simulink model "matlab_file_rl"  (R2018a)
settings: Solver=FixedStepAuto  StartTime=0.0  StopTime=1  RelTol=1e-3
libraries: androiduilib x4
settings Model: Creator=akshay  LastModifiedBy=akshay
settings DataIOCC: LimitDataPoints=on  MaxDataPoints=5000
settings OptimizationCC: EnhancedBackFolding=on  PassReuseOutputArgsAs=Individual arguments  MaxStackSize=64  OptimizeBlockOrder=speed  DifferentSizesBufferReuse=on  OptimizationCustomize=off
settings DebuggingCC: ParameterTunabilityLossMsg=error
settings HardwareCC: ProdBitPerPointer=32  ProdBitPerSizeT=32  ProdBitPerPtrDiffT=32  ProdLargestAtomicInteger=Long  ProdLargestAtomicFloat=Double  ProdWordSize=32  ProdHWDeviceType=ARM Compatible->ARM Cortex
settings SFSimCC: MATLABDynamicMemAlloc=off
settings RTWCC: SystemTargetFile=ert.tlc  HardwareBoard=Android Device  TLCOptions="-aInlineSetEventsForThisBaseRateFcn=TLC_FALSE -aSuppressMultiTaskScheduler=TLC_FALSE  -aRateBasedStepFcn=0"  TemplateMakefile=ert_default_tmf  GenerateReport=on  RTWVerbose=off  Toolchain=Android SDK/NDK Tools  BuildConfiguration=Faster Runs  IncludeHyperlinkInReport=on  LaunchReport=on  GenerateTraceInfo=on  GenerateTraceReport=on  GenerateTraceReportSl=on  GenerateTraceReportSf=on  GenerateTraceReportEml=on
settings CodeAppCC: ForceParamTrailComments=on  IgnoreCustomStorageClasses=off  OperatorAnnotations=on  SimulinkDataObjDesc=on  SFDataObjDesc=on  InsertBlockDesc=on

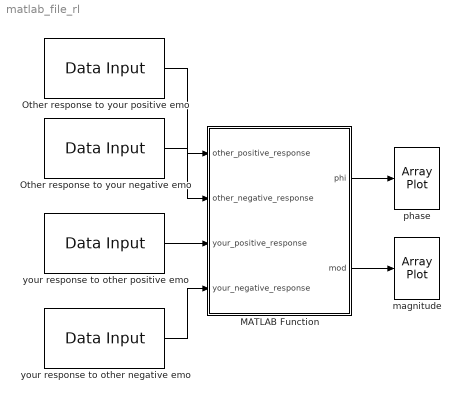
== system matlab_file_rl ==
  MATLAB Function : MATLAB Function  TreatAsAtomicUnit=on
  Other response to your negative emo : androiduilib/Data Input  isCharVector=off  Value=1  CharVector=Hello World  OutputDataType=double  maxCharVectorSize=100  DataInputId=matlab_file_rl/Other_response_to_your_negative_emo  SampleTime=0.1
      settings: SourceProductName=Simulink Support Package for Android Devices  SourceProductBaseCode=ANDROID
  Other response to your positive emo : androiduilib/Data Input  isCharVector=off  Value=1  CharVector=Hello World  OutputDataType=double  maxCharVectorSize=100  DataInputId=matlab_file_rl/Other_response_to_your_positive_emo  SampleTime=0.1
      settings: SourceProductName=Simulink Support Package for Android Devices  SourceProductBaseCode=ANDROID
  magnitude : ArrayPlot
  phase : ArrayPlot
  your response to other negative emo : androiduilib/Data Input  isCharVector=off  Value=1.0  CharVector=Hello World  OutputDataType=double  maxCharVectorSize=100  DataInputId=matlab_file_rl/your_response_to_other_negative_emo  SampleTime=0.1
      settings: SourceProductName=Simulink Support Package for Android Devices  SourceProductBaseCode=ANDROID
  your response to other positive emo : androiduilib/Data Input  isCharVector=off  Value=1.0  CharVector=Hello World  OutputDataType=double  maxCharVectorSize=100  DataInputId=matlab_file_rl/your_response_to_other_positive_emo  SampleTime=0.1
      settings: SourceProductName=Simulink Support Package for Android Devices  SourceProductBaseCode=ANDROID
  wires:
  Other response to your negative emo/1 -> MATLAB Function/2(other_negative_response)
  Other response to your positive emo/1 -> MATLAB Function/1(other_positive_response)
  your response to other positive emo/1 -> MATLAB Function/3(your_positive_response)
  your response to other negative emo/1 -> MATLAB Function/4(your_negative_response)
  MATLAB Function/1(phi) -> phase/1
  MATLAB Function/2(mod) -> magnitude/1

== matlab function matlab_file_rl/MATLAB Function ==
  data: other_positive_response input; phi output; other_negative_response input; your_positive_response input; your_negative_response input; mod output
function [phi, mod]  = rl_relation(other_positive_response,other_negative_response,...
    your_positive_response,your_negative_response)
[x,y] = meshgrid(-8:0.2:8,-8:0.2:8);
% asking question
% explain behavior of partner
% logic questions
% other_positive_response=input('others reponse to your positive feeling');
% other_negative_response=input('others reponse to your negative feeling');
% your_positive_response= input('your response to others positive feeling');
% your_negative_response= input('your response to others negative feeling');
% 2^4 functions


% 1 represents + ve emotions
% u= x
% v=y
% 0000 0001 0010 0011 0100 0101 0110 0111 1000 1001 1010 1011 1100 1101 1110 1111
%1 1111
if other_positive_response ==1 && other_negative_response== 1 &&...
your_positive_response== 1 && your_negative_response==1
u= y.^2;
v= x.^2;
w= u+j.*v;
out_1=reshape(u,length(u)*length(u),1);
out_2=reshape(v,length(v)*length(v),1);
out=reshape(w,length(w)*length(w),1);
phi= rad2deg(angle(out));
mod= abs(out);
%2 1110
elseif other_positive_response ==1 && other_negative_response== 1 &&...
your_positive_response== 1 && your_negative_response==0
u= y.^3;
v= x.^2;
w= u+j.*v;
out_1=reshape(u,length(u)*length(u),1);
out_2=reshape(v,length(v)*length(v),1);
out=reshape(w,length(w)*length(w),1);  
phi= rad2deg(angle(out));
mod= abs(out);    
%3 1101
elseif other_positive_response ==1 && other_negative_response== 1 &&...
your_positive_response== 0 && your_negative_response==1
u= -y.^3;
v= x.^2;
w= u+j.*v;
out_1=reshape(u,length(u)*length(u),1);
out_2=reshape(v,length(v)*length(v),1);
out=reshape(w,length(w)*length(w),1);
phi= rad2deg(angle(out));
mod= abs(out);
%4 1100
elseif other_positive_response ==1 && other_negative_response== 1 &&...
your_positive_response== 0 && your_negative_response==0
u= -y.^2;
v= x.^2;
w= u+j.*v;
out_1=reshape(u,length(u)*length(u),1);
out_2=reshape(v,length(v)*length(v),1);
out=reshape(w,length(w)*length(w),1);
phi= rad2deg(angle(out));
mod= abs(out);
%5 1011
elseif other_positive_response ==1 && other_negative_response== 0 &&...
your_positive_response== 1 && your_negative_response==1
u= y.^2;
v= x.^3;
w= u+j.*v;
out_1=reshape(u,length(u)*length(u),1);
out_2=reshape(v,length(v)*length(v),1);
out=reshape(w,length(w)*length(w),1);
phi= rad2deg(angle(out));
mod= abs(out);
%6 1010
elseif other_positive_response ==1 && other_negative_response== 0 &&...
your_positive_response== 1 && your_negative_response==0
u= y.^3;
v= x.^3;
w= u+j.*v;
out_1=reshape(u,length(u)*length(u),1);
out_2=reshape(v,length(v)*length(v),1);
out=reshape(w,length(w)*length(w),1);
phi= rad2deg(angle(out));
mod= abs(out);
%7 1001 other respond positive to your positive & negative to negative
% you respond -ve to their +ve and +ve to their -ve 
elseif other_positive_response ==1 && other_negative_response== 0 &&...
your_positive_response== 0 && your_negative_response==1
u= -y.^3;
v= x.^3;
w= u+j.*v;
out_1=reshape(u,length(u)*length(u),1);
out_2=reshape(v,length(v)*length(v),1);
out=reshape(w,length(w)*length(w),1);
phi= rad2deg(angle(out));
mod= abs(out);
% 8 1000
elseif other_positive_response ==1 && other_negative_response== 0 &&...
your_positive_response== 0 && your_negative_response==0
u= -y.^2;
v= x.^3;
w= u+j.*v;
out_1=reshape(u,length(u)*length(u),1);
out_2=reshape(v,length(v)*length(v),1);
out=reshape(w,length(w)*length(w),1);
phi= rad2deg(angle(out));
mod= abs(out);
%9 0111
elseif other_positive_response ==0 && other_negative_response== 1 &&...
your_positive_response==1 && your_negative_response==1
u= +y.^2;
v= -x.^3;
w= u+j.*v;
out_1=reshape(u,length(u)*length(u),1);
out_2=reshape(v,length(v)*length(v),1);
out=reshape(w,length(w)*length(w),1);
phi= rad2deg(angle(out));
mod= abs(out);
%10 0110
elseif other_positive_response ==0 && other_negative_response== 1 &&...
your_positive_response== 1 && your_negative_response==0
u= y.^3;
v= -x.^3;
w= u+j.*v;
out_1=reshape(u,length(u)*length(u),1);
out_2=reshape(v,length(v)*length(v),1);
out=reshape(w,length(w)*length(w),1);
phi= rad2deg(angle(out));
mod= abs(out);
% 11 0101
elseif other_positive_response ==0 && other_negative_response== 1 &&...
your_positive_response== 0 && your_negative_response==1
u= -y.^3;
v= -x.^3;
w= u+j.*v;
out_1=reshape(u,length(u)*length(u),1);
out_2=reshape(v,length(v)*length(v),1);
out=reshape(w,length(w)*length(w),1);
phi= rad2deg(angle(out));
mod= abs(out);
% 12 0100
elseif other_positive_response ==0 && other_negative_response== 1 &&...
your_positive_response== 0 && your_negative_response==0
u= -y.^2;
v= -x.^3;
w= u+j.*v;
out_1=reshape(u,length(u)*length(u),1);
out_2=reshape(v,length(v)*length(v),1);
out=reshape(w,length(w)*length(w),1);
phi= rad2deg(angle(out));
mod= abs(out);
% 13 0011
elseif other_positive_response ==0 && other_negative_response== 0 &&...
your_positive_response== 1 && your_negative_response==1
u= y.^2;
v= -x.^2;
w= u+j.*v;
out_1=reshape(u,length(u)*length(u),1);
out_2=reshape(v,length(v)*length(v),1);
out=reshape(w,length(w)*length(w),1);
phi= rad2deg(angle(out));
mod= abs(out);
% 14 0010
elseif other_positive_response ==0 && other_negative_response==0 &&...
your_positive_response== 1 && your_negative_response==0
u= y.^3;
v= -x.^2;
w= u+j.*v;
out_1=reshape(u,length(u)*length(u),1);
out_2=reshape(v,length(v)*length(v),1);
out=reshape(w,length(w)*length(w),1);
phi= rad2deg(angle(out));
mod= abs(out);
% 15 0001
elseif other_positive_response ==0 && other_negative_response== 0 &&...
your_positive_response== 0 && your_negative_response==1
u= -y.^3;
v= -x.^2;
w= u+j.*v;
out_1=reshape(u,length(u)*length(u),1);
out_2=reshape(v,length(v)*length(v),1);
out=reshape(w,length(w)*length(w),1);
phi= rad2deg(angle(out));
mod= abs(out);
% 16 0000
elseif other_positive_response ==0 && other_negative_response== 0 &&...
your_positive_response== 0 && your_negative_response==0
u= -y.^2;
v= -x.^2;
w= u+j.*v;
out_1=reshape(u,length(u)*length(u),1);
out_2=reshape(v,length(v)*length(v),1);
out=reshape(w,length(w)*length(w),1);
phi= rad2deg(angle(out));
mod= abs(out);
else 
u = (y-x)*x-(y-x)*y;
v = (x-y)*y-(x-y)*x;
w= u+j.*v;
out_1=reshape(u,length(u)*length(u),1);
out_2=reshape(v,length(v)*length(v),1);
out=reshape(w,length(w)*length(w),1);
phi= rad2deg(angle(out));
mod= abs(out);
end
% figure
% quiver(x,y,u,v)
